simulink model "RCAMSimProj"  (R2023b)
settings: Solver=VariableStepAuto  StartTime=0.0  StopTime=TF  RelTol=1e-3
values from neighbouring files (symbols this model uses):
  h0 = 1000    [RCAMSimulationProj.m]
  lambda0 = deg2rad(122.3075)    [RCAMSimulationProj.m]
  phi0 = deg2rad(47.6546)    [RCAMSimulationProj.m]
  u1max = 25*pi/180    (= 0.436332312999)    [RCAMSimulationProj.m]
  u1min = -25*pi/180    (= -0.436332312999)    [RCAMSimulationProj.m]
  u2max = 25*pi/180    (= 0.436332312999)    [RCAMSimulationProj.m]
  u2min = -25*pi/180    (= -0.436332312999)    [RCAMSimulationProj.m]
  u3max = 30*pi/180    (= 0.523598775598)    [RCAMSimulationProj.m]
  u3min = -30*pi/180    (= -0.523598775598)    [RCAMSimulationProj.m]
  u4max = 1000*pi/180    (= 17.4532925199)    [RCAMSimulationProj.m]
  u4min = 0.5*pi/180    (= 0.00872664625997)    [RCAMSimulationProj.m]
  u5max = 1000*pi/180    (= 17.4532925199)    [RCAMSimulationProj.m]
  u5min = 0.5*pi/180    (= 0.00872664625997)    [RCAMSimulationProj.m]
  x0 = [84.9985000000000;0;0.504800000000000;0;0;0;0;0.00590000000000000;0]    [RCAMSimulationProj.m]
undefined symbols (not defined in the file or in its folder): navigation_eqn, RCAM_model, trimProj
libraries: aerolibfltsims x2, aerolibanimutils x1
settings Model: Creator=ahmed  LastModifiedBy=ahmed

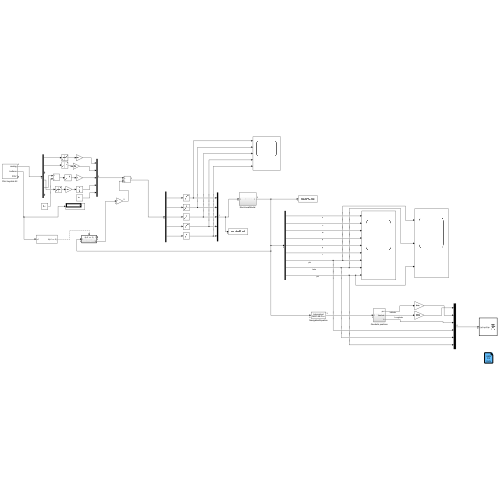
[thumbnail: Simulink's stored preview of the top-level diagram]
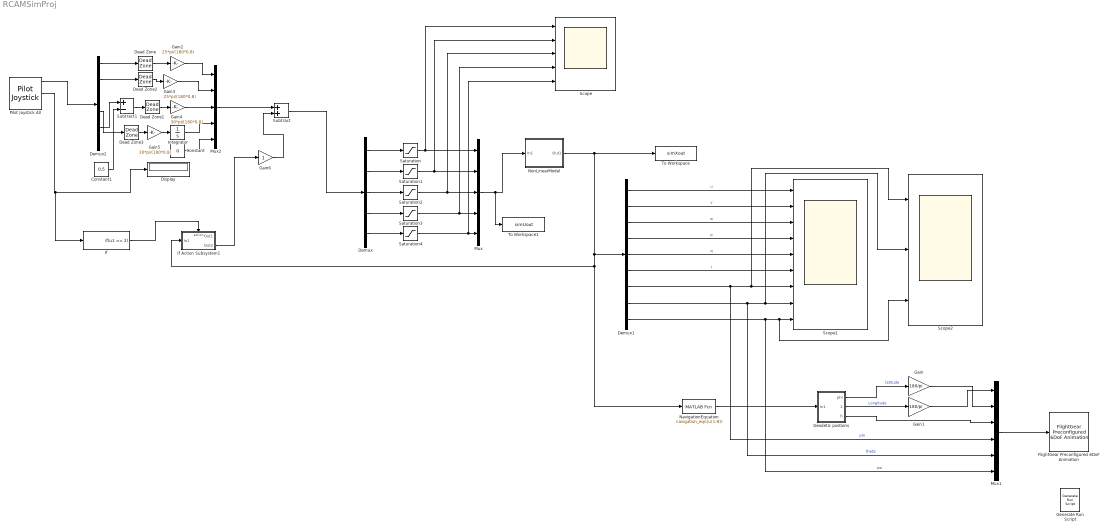
== system RCAMSimProj ==
  Constant : Constant  Value=0
  Constant1 : Constant  Value=0.5
  Dead Zone{,1..3} (4 alike) : DeadZone  LowerValue=-0.2  UpperValue=0.2
  Demux : Demux  Outputs=5
  Demux1 : Demux  Outputs=9
  Demux2 : Demux  Outputs=6
  Display : Display
  FlightGear Preconfigured 6DoF Animation : aerolibfltsims/FlightGear Preconfigured 6DoF Animation  xFlightGearVersion=v2019.1  DestinationIpAddress=127.0.0.1  DestinationPort=5502  SampleTime=1/30  packetVersion=24
  Gain : Gain  Gain=180/pi
  Gain1 : Gain  Gain=180/pi
  Gain2 : Gain  Gain=25*pi/(180*0.8)
  Gain3 : Gain  Gain=25*pi/(180*0.8)
  Gain4 : Gain  Gain=30*pi/(180*0.8)
  Gain5 : Gain  Gain=30*pi/(180*0.8)
  Gain6 : Gain
  Generate Run Script : aerolibfltsims/Generate Run Script  Architecture=Win64  dataFlow=Send  GeometryModelName=c172p  AirportId=KSFO  RunwayId=10L  InitialAltitude=7224  InitialHeading=113  OffsetDistance=4.72  OffsetAzimuth=0  InstallScenery=on  DisableShaders=on  OriginAddress=127.0.0.1  DestinationPort=5502  OriginPort=5505  LocalAddress=127.0.0.1  OutputFileName=runfg.bat  FlightGearBaseDirectory=D:\Program Files\FlightGear 2020.3
  Geodetic postions : Subsystem
  If : If  IfExpression=u1 == 2  ShowElse=off
  If Action Subsystem1 : Subsystem  TreatAsAtomicUnit=on
  Integrator : Integrator
  Mux : Mux  Inputs=5
  Mux1 : Mux  Inputs=6
  Mux2 : Mux  Inputs=5
  NavigationEquation : MATLABFcn  MATLABFcn=navigation_eqn(u(1:9))
  NonLinearModel : Subsystem
  Pilot Joystick All : aerolibanimutils/Pilot Joystick  JoystickID=Joystick1  OutputConfiguration=AllOutputs  SampleTime=1/30
      settings: LibrarySourceBlock=aerolibanimutils/Pilot Joystick All
  Saturation : Saturate  UpperLimit=u1max  LowerLimit=u1min
  Saturation1 : Saturate  UpperLimit=u2max  LowerLimit=u2min
  Saturation2 : Saturate  UpperLimit=u3max  LowerLimit=u3min
  Saturation3 : Saturate  UpperLimit=u4max  LowerLimit=u4min
  Saturation4 : Saturate  UpperLimit=u5max  LowerLimit=u5min
  Scope : Scope  NumInputPorts=5
  Scope1 : Scope  NumInputPorts=9
  Scope2 : Scope  NumInputPorts=3
  Subtract : Sum
  Subtract1 : Sum  Inputs=+-
  To Workspace : ToWorkspace  VariableName=simXout  SaveFormat=Timeseries  SampleTime=-1
  To Workspace1 : ToWorkspace  VariableName=simUout  SaveFormat=Timeseries  SampleTime=-1
  wires:
  Demux/1 -> Saturation/1
  Demux/2 -> Saturation1/1
  Demux/3 -> Saturation2/1
  Demux/4 -> Saturation3/1
  Demux/5 -> Saturation4/1
  Saturation3/1 -> Mux/4, Scope/4
  Mux/1 -> To Workspace1/1, NonLinearModel/1(In1)
  Saturation/1 -> Scope/1, Mux/1
  Saturation4/1 -> Scope/5, Mux/5
  Saturation2/1 -> Scope/3, Mux/3
  Saturation1/1 -> Scope/2, Mux/2
  Subtract/1 -> Demux/1
  Demux1/1 -> Scope1/1  "u"
  Demux1/2 -> Scope1/2  "v"
  Demux1/3 -> Scope1/3  "w"
  Demux1/4 -> Scope1/4  "p"
  Demux1/5 -> Scope1/5  "q"
  Demux1/6 -> Scope1/6  "r"
  Demux1/7 -> Mux1/4, Scope2/1, Scope1/7  "phi"
  Demux1/8 -> Mux1/5, Scope2/2, Scope1/8  "theta"
  Demux1/9 -> Mux1/6, Scope2/3, Scope1/9  "psi"
  NavigationEquation/1 -> Geodetic postions/1(In1)
  Geodetic postions/1(phi) -> Gain/1  "latitude"
  Geodetic postions/2(lambda) -> Gain1/1  "Longitude"
  Geodetic postions/3(h) -> Mux1/3
  Gain1/1 -> Mux1/1
  Gain/1 -> Mux1/2
  Mux1/1 -> FlightGear Preconfigured 6DoF Animation/1
  Demux2/1 -> Dead Zone/1
  Demux2/2 -> Dead Zone2/1
  Gain4/1 -> Mux2/3
  Gain3/1 -> Mux2/2
  Gain2/1 -> Mux2/1
  Gain5/1 -> Integrator/1
  Pilot Joystick All/1 -> Demux2/1
  Dead Zone/1 -> Gain2/1
  Dead Zone2/1 -> Gain3/1
  Dead Zone3/1 -> Gain5/1
  Dead Zone1/1 -> Gain4/1
  Pilot Joystick All/2 -> Display/1, If/1
  Mux2/1 -> Subtract/1
  If/1 -> If Action Subsystem1/Action
  If Action Subsystem1/2(Out2) -> Gain6/1
  Gain6/1 -> Subtract/2
  Demux2/4 -> Dead Zone3/1
  Constant1/1 -> Subtract1/2
  Demux2/5 -> Subtract1/1
  Subtract1/1 -> Dead Zone1/1
  NonLinearModel/1(Out1) -> If Action Subsystem1/1(In1), NavigationEquation/1, Demux1/1, To Workspace/1
  Integrator/1 -> Mux2/4
  Constant/1 -> Mux2/5

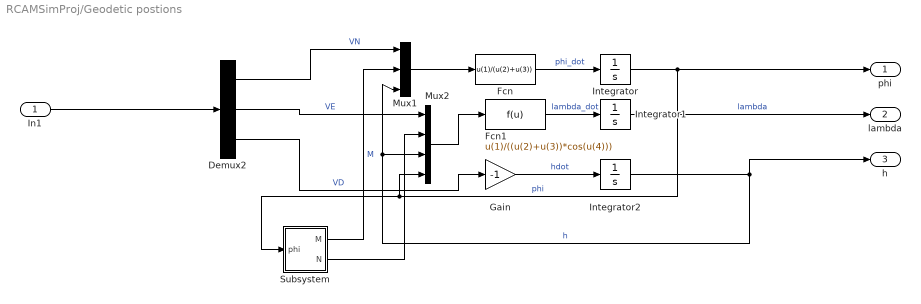
== system RCAMSimProj/Geodetic postions ==
  In1 : Inport
  Demux2 : Demux  Outputs=3
  Fcn : Fcn  Expr=u(1)/(u(2)+u(3))
  Fcn1 : Fcn  Expr=u(1)/((u(2)+u(3))*cos(u(4)))
  Gain : Gain  Gain=-1
  Integrator : Integrator  InitialCondition=phi0
  Integrator1 : Integrator  InitialCondition=lambda0
  Integrator2 : Integrator  InitialCondition=h0
  Mux1 : Mux  Inputs=3
  Mux2 : Mux
  Subsystem : Subsystem
  phi : Outport
  lambda : Outport  Port=2
  h : Outport  Port=3
  wires:
  Integrator2/1 -> h/1, Mux2/3, Mux1/3  "h"
  Fcn1/1 -> Integrator1/1  "lambda_dot"
  Gain/1 -> Integrator2/1  "hdot"
  Demux2/3 -> Gain/1  "VD"
  Demux2/2 -> Mux2/1  "VE"
  Integrator/1 -> phi/1, Mux2/4, Subsystem/1(phi)  "phi"
  Subsystem/2(N) -> Mux2/2
  Fcn/1 -> Integrator/1  "phi_dot"
  Subsystem/1(M) -> Mux1/2  "M"
  Demux2/1 -> Mux1/1  "VN"
  Mux1/1 -> Fcn/1
  Mux2/1 -> Fcn1/1
  Integrator1/1 -> lambda/1  "lambda"
  In1/1 -> Demux2/1

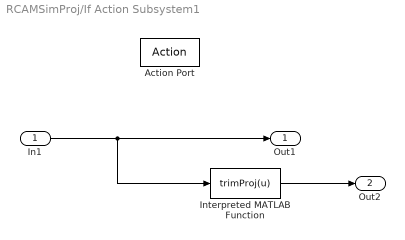
== system RCAMSimProj/If Action Subsystem1 ==
  In1 : Inport
  Action Port : ActionPort  ActionPortLabel=if(u1 == 2)
  Interpreted MATLAB Function : MATLABFcn  MATLABFcn=trimProj(u)
  Out1 : Outport
  Out2 : Outport  Port=2
  wires:
  In1/1 -> Interpreted MATLAB Function/1, Out1/1
  Interpreted MATLAB Function/1 -> Out2/1

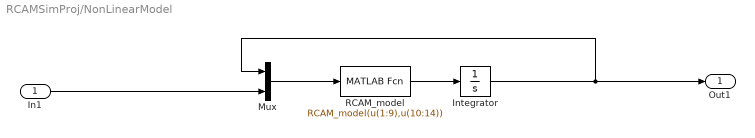
== system RCAMSimProj/NonLinearModel ==
  In1 : Inport
  Integrator : Integrator  InitialCondition=x0
  Mux : Mux  Inputs=2
  RCAM_model : MATLABFcn  MATLABFcn=RCAM_model(u(1:9),u(10:14))
  Out1 : Outport
  wires:
  RCAM_model/1 -> Integrator/1
  Mux/1 -> RCAM_model/1
  Integrator/1 -> Mux/1, Out1/1
  In1/1 -> Mux/2

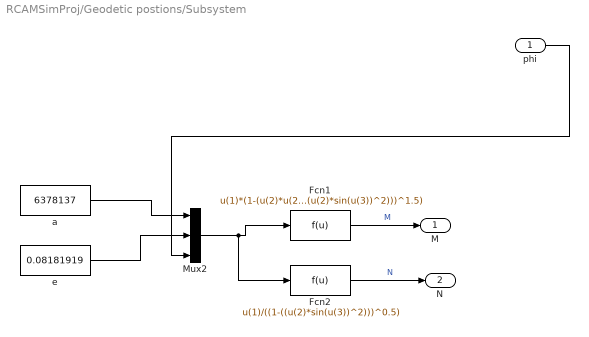
== system RCAMSimProj/Geodetic postions/Subsystem ==
  phi : Inport
  Fcn1 : Fcn  Expr=u(1)*(1-(u(2)*u(2)))/((1-((u(2)*sin(u(3))^2)))^1.5)
  Fcn2 : Fcn  Expr=u(1)/((1-((u(2)*sin(u(3))^2)))^0.5)
  Mux2 : Mux  Inputs=3
  a : Constant  Value=6378137
  e : Constant  Value=0.08181919
  M : Outport
  N : Outport  Port=2
  wires:
  Mux2/1 -> Fcn2/1, Fcn1/1
  Fcn1/1 -> M/1  "M"
  phi/1 -> Mux2/3
  a/1 -> Mux2/1
  e/1 -> Mux2/2
  Fcn2/1 -> N/1  "N"
